simulink model "RBDmodel_unprotected"  (R2023a)
settings: Solver=ode15s  StartTime=0.0  StopTime=10  FixedStep=0.0001  RelTol=1e-3  AbsTol=1e-3  EnableMultiTasking=on
model workspace (MAT data in the model file):
  C_Gimbal = 0.1
  C_IAP = 0.01
  IAP_Pa = 0
  K_Gimbal = 0
  K_IAP = 0
  Left_EO = 0
  Left_IO = 0
  Left_MF = 0
  Left_RA = 0
  Moment_AR = 0
  Moment_FE = 7.5
  Moment_LB = 0
  Right_EO = 0
  Right_IO = 0
  Right_MF = 0
  Right_RA = 0
  a = 1
  b = 1
  muscle_color = [0 0 1]
  muscle_radius = 1
undefined symbols (not defined in the file): X, Y, Z
libraries: nesl_utility x346, sm_lib x329, simulink_extras x33, checkpacklib x3, simulink x1
(part 1 of 13)
settings Model: PacingRate=0.110000  Creator=Siril TD  LastModifiedBy=siril
settings SolverCC: ZeroCrossAlgorithm=Adaptive  AutoInsertRateTranBlk=on
settings DataIOCC: LimitDataPoints=on  MaxDataPoints=50000  ReturnWorkspaceOutputsName=SDOSimTest_Log
settings OptimizationCC: LifeSpan=inf
settings DebuggingCC: IgnoredZcDiagnostic=none  UnconnectedInputMsg=warning  UnconnectedOutputMsg=warning  UnconnectedLineMsg=warning  AllowSymbolicDim=off  SFUnexpectedBacktrackingDiag=warning  SFNoUnconditionalDefaultTransitionDiag=warning  SFExecutionAtInitializationDiag=none  ArithmeticOperatorsInVariantConditions=warning
settings ModelReferenceCC: EnableRefExpFcnMdlSchedulingChecks=on
settings SFSimCC: SimUseLocalCustomCode=off  CustomCodeUndefinedFunction=UseInterfaceOnly
settings RTWCC: RTWUseLocalCustomCode=off  DLArmComputeVersion=19.05
settings CodeAppCC: StateflowObjectComments=on
settings GRTTargetCC: TargetLangStandard=C89/C90 (ANSI)
settings ConfigComp: CovMetricSettings=dw  CovSaveCumulativeToWorkspaceVar=on  CovSaveSingleToWorkspaceVar=on  CovExternalEMLEnable=off  CovSFcnEnable=off
settings SimscapeCC: SimscapeLogType=all  SimscapeLogSimulationStatistics=on  SimscapeLogDataHistory=10000

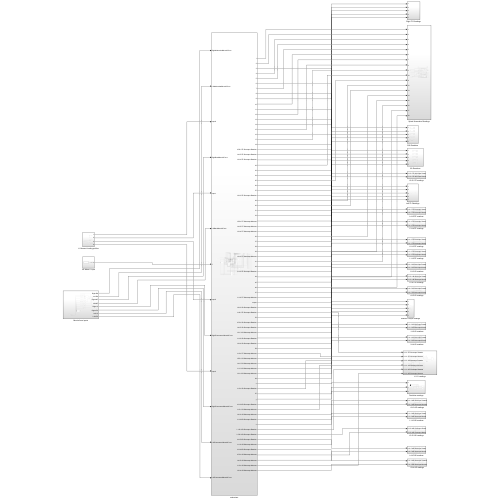
[thumbnail: Simulink's stored preview of the top-level diagram]
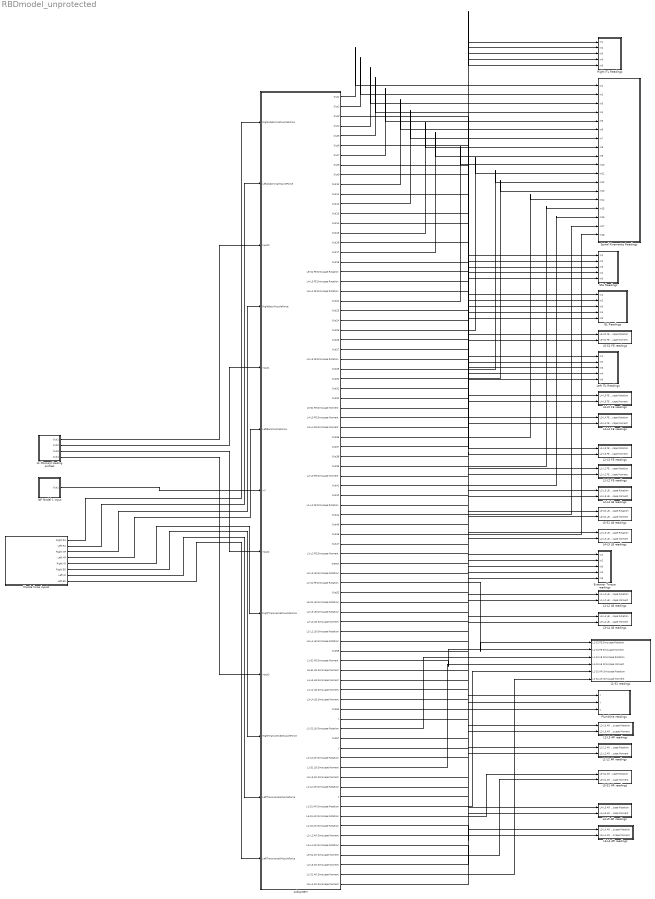
== system RBDmodel_unprotected ==
  Extensor Torque readings : Subsystem
  IAP Model 1 input : Subsystem
  ISL Readings : Subsystem
  L1 Moment loading profiles : Subsystem
  L1-L2 AR readings : Subsystem
  L1-L2 FE readings : Subsystem
  L1-L2 LB readings : Subsystem
  L1-S1 readings : Subsystem
  L2-L3 AR readings : Subsystem
  L2-L3 FE readings : Subsystem
  L2-L3 LB readings : Subsystem
  L3-L4 AR readings : Subsystem
  L3-L4 FE readings : Subsystem
  L3-L4 LB readings : Subsystem
  L4-L5 AR readings : Subsystem
  L4-L5 FE readings : Subsystem
  L4-L5 LB readings : Subsystem
  L5-S1 AR readings : Subsystem
  L5-S1 FE readings : Subsystem
  L5-S1 LB readings : Subsystem
  Left ITL Readings : Subsystem
  Muscle force inputs : Subsystem
  Plumbline readings : Subsystem
  Right ITL Readings : Subsystem
  SSL Readings : Subsystem
  Spinal Kinematics Readings : Subsystem
  subsystem : Subsystem
  wires:
  Muscle force inputs/1(Right RA) -> subsystem/1(RightAbdominalMuscleForce)
  Muscle force inputs/2(Left RA) -> subsystem/2(LeftAbdominalMuscleForce)
  L1 Moment loading profiles/1(Out1) -> subsystem/3(input0)
  Muscle force inputs/3(Right MF) -> subsystem/4(RightBackMuscleForce)
  L1 Moment loading profiles/2(Out2) -> subsystem/5(input1)
  Muscle force inputs/4(Left MF) -> subsystem/6(LeftBackMuscleForce)
  IAP Model 1 input/1(Out1) -> subsystem/7(In7)
  L1 Moment loading profiles/3(Out3) -> subsystem/8(input2)
  Muscle force inputs/5(Right IO) -> subsystem/9(RightTransverse1MuscleForce)
  L1 Moment loading profiles/4(Out4) -> subsystem/10(input3)
  Muscle force inputs/6(Right EO) -> subsystem/11(RightTransverse2MuscleForce)
  Muscle force inputs/7(Left IO) -> subsystem/12(LeftTransverse1MuscleForce)
  Muscle force inputs/8(Left EO) -> subsystem/13(LeftTransverse2MuscleForce)
  subsystem/1(Out1) -> Spinal Kinematics Readings/1(In1)
  subsystem/2(Out2) -> Spinal Kinematics Readings/2(In2)
  subsystem/3(Out3) -> ISL Readings/1(In1)
  subsystem/4(Out4) -> Spinal Kinematics Readings/3(In3)
  subsystem/5(Out5) -> Spinal Kinematics Readings/4(In4)
  subsystem/6(Out6) -> SSL Readings/1(In1)
  subsystem/7(Out7) -> Spinal Kinematics Readings/5(In5)
  subsystem/8(Out8) -> Left ITL Readings/1(In1)
  subsystem/9(Out9) -> Right ITL Readings/1(In1)
  subsystem/10(Out10) -> Spinal Kinematics Readings/6(In6)
  subsystem/11(Out11) -> ISL Readings/2(In2)
  subsystem/12(Out12) -> Spinal Kinematics Readings/7(In7)
  subsystem/13(Out13) -> SSL Readings/2(In2)
  subsystem/14(Out14) -> Right ITL Readings/2(In2)
  subsystem/15(Out15) -> Spinal Kinematics Readings/8(In8)
  subsystem/16(Out16) -> Left ITL Readings/2(In2)
  subsystem/17(Out17) -> Spinal Kinematics Readings/9(In9)
  subsystem/18(Out18) -> Right ITL Readings/3(In3)
  subsystem/19(L5-S1 FE Simscape Rotation) -> L5-S1 FE readings/1(L5-S1 FE Simscape Rotation)
  subsystem/20(L4-L5 FE Simscape Rotation) -> L4-L5 FE readings/1(L4-L5 FE Simscape Rotation)
  subsystem/21(L3-L4 FE Simscape Rotation) -> L3-L4 FE readings/1(L3-L4 FE Simscape Rotation)
  subsystem/22(Out22) -> Spinal Kinematics Readings/10(In10)
  subsystem/23(Out23) -> ISL Readings/3(In3)
  subsystem/24(Out24) -> SSL Readings/3(In3)
  subsystem/25(Out25) -> Spinal Kinematics Readings/11(In11)
  subsystem/26(Out26) -> Left ITL Readings/3(In3)
  subsystem/27(Out27) -> Right ITL Readings/4(In4)
  subsystem/28(L2-L3 FE Simscape Rotation) -> L2-L3 FE readings/1(L2-L3 FE Simscape Rotation)
  subsystem/29(Out29) -> Spinal Kinematics Readings/12(In12)
  subsystem/30(Out30) -> Spinal Kinematics Readings/13(In13)
  subsystem/31(Out31) -> SSL Readings/4(In4)
  subsystem/32(Out32) -> Right ITL Readings/5(In5)
  subsystem/33(L5-S1 FE Simscape Moment) -> L5-S1 FE readings/2(L5-S1 FE Simscape Moment)
  subsystem/34(L4-L5 FE Simscape Moment) -> L4-L5 FE readings/2(L4-L5 FE Simscape Moment)
  subsystem/35(L3-L4 FE Simscape Moment) -> L3-L4 FE readings/2(L3-L4 FE Simscape Moment)
  subsystem/36(Out36) -> Spinal Kinematics Readings/14(In14)
  subsystem/37(Out37) -> ISL Readings/4(In4)
  subsystem/38(Out38) -> Left ITL Readings/4(In4)
  subsystem/39(Out39) -> Spinal Kinematics Readings/15(In15)
  subsystem/40(L2-L3 FE Simscape Moment) -> L2-L3 FE readings/2(L2-L3 FE Simscape Moment)
  subsystem/41(Out41) -> Spinal Kinematics Readings/16(In16)
  subsystem/42(Out42) -> SSL Readings/5(In5)
  subsystem/43(L1-L2 FE Simscape Rotation) -> L1-L2 FE readings/1(L1-L2 FE Simscape Rotation)
  subsystem/44(Out44) -> Spinal Kinematics Readings/17(In17)
  subsystem/45(Out45) -> Left ITL Readings/5(In5)
  subsystem/46(Out46) -> Spinal Kinematics Readings/18(In18)
  subsystem/47(Out47) -> ISL Readings/5(In5)
  subsystem/48(L1-L2 FE Simscape Moment) -> L1-L2 FE readings/2(L1-L2 FE Simscape Moment)
  subsystem/49(output) -> Extensor Torque readings/1(In1)
  subsystem/50(L2-L3 LB Simscape Rotation) -> L2-L3 LB readings/1(L2-L3 LB Simscape Rotation)
  subsystem/51(L1-S1 FE Simscape Rotation) -> L1-S1 readings/1(L1-S1 FE Simscape Rotation)
  subsystem/52(Out52) -> Extensor Torque readings/2(In2)
  subsystem/53(L5-S1 LB Simscape Rotation) -> L5-S1 LB readings/1(L5-S1 LB Simscape Rotation)
  subsystem/54(L4-L5 LB Simscape Rotation) -> L4-L5 LB readings/1(L4-L5 LB Simscape Rotation)
  subsystem/55(L2-L3 LB Simscape Moment) -> L2-L3 LB readings/2(L2-L3 LB Simscape Moment)
  subsystem/56(L1-L2 LB Simscape Rotation) -> L1-L2 LB readings/1(L1-L2 LB Simscape Rotation)
  subsystem/57(L3-L4 LB Simscape Rotation) -> L3-L4 LB readings/1(L3-L4 LB Simscape Rotation)
  subsystem/58(Out58) -> Extensor Torque readings/3(In3)
  subsystem/59(L1-S1 FE Simscape Moment) -> L1-S1 readings/2(L1-S1 FE Simscape Moment)
  subsystem/60(L5-S1 LB Simscape Moment) -> L5-S1 LB readings/2(L5-S1 LB Simscape Moment)
  subsystem/61(L4-L5 LB Simscape Moment) -> L4-L5 LB readings/2(L4-L5 LB Simscape Moment)
  subsystem/62(L1-L2 LB Simscape Moment) -> L1-L2 LB readings/2(L1-L2 LB Simscape Moment)
  subsystem/63(L3-L4 LB Simscape Moment) -> L3-L4 LB readings/2(L3-L4 LB Simscape Moment)
  subsystem/64(Out64) -> Extensor Torque readings/4(In4)
  subsystem/65(x) -> Plumbline readings/1(x)
  subsystem/66(L1-S1 LB Simscape Rotation) -> L1-S1 readings/3(L1-S1 LB Simscape Rotation)
  subsystem/67(Out67) -> Extensor Torque readings/5(In5)
  subsystem/68(y) -> Plumbline readings/2(y)
  subsystem/69(L2-L3 AR Simscape Rotation) -> L2-L3 AR readings/1(L2-L3 AR Simscape Rotation)
  subsystem/70(L1-S1 LB Simscape Moment) -> L1-S1 readings/4(L1-S1 LB Simscape Moment)
  subsystem/71(L2-L3 AR Simscape Moment) -> L2-L3 AR readings/2(L2-L3 AR Simscape Moment)
  subsystem/72(L1-L2 AR Simscape Rotation) -> L1-L2 AR readings/1(L1-L2 AR Simscape Rotation)
  subsystem/73(z) -> Plumbline readings/3(z)
  subsystem/74(L1-S1 AR Simscape Rotation) -> L1-S1 readings/5(L1-S1 AR Simscape Rotation)
  subsystem/75(L5-S1 AR Simscape Rotation) -> L5-S1 AR readings/1(L5-S1 AR Simscape Rotation)
  subsystem/76(L4-L5 AR Simscape Rotation) -> L4-L5 AR readings/1(L4-L5 AR Simscape Rotation)
  subsystem/77(L1-L2 AR Simscape Moment) -> L1-L2 AR readings/2(L1-L2 AR Simscape Moment)
  subsystem/78(L3-L4 AR Simscape Rotation) -> L3-L4 AR readings/1(L3-L4 AR Simscape Rotation)
  subsystem/79(L5-S1 AR Simscape Moment) -> L5-S1 AR readings/2(L5-S1 AR Simscape Moment)
  subsystem/80(L4-L5 AR Simscape Moment) -> L4-L5 AR readings/2(L4-L5 AR Simscape Moment)
  subsystem/81(L1-S1 AR Simscape Moment) -> L1-S1 readings/6(L1-S1 AR Simscape Moment)
  subsystem/82(L3-L4 AR Simscape Moment) -> L3-L4 AR readings/2(L3-L4 AR Simscape Moment)

== system RBDmodel_unprotected/Extensor Torque readings ==
  In1 : Inport
  In2 : Inport  Port=2
  In3 : Inport  Port=3
  In4 : Inport  Port=4
  In5 : Inport  Port=5
  Display{,1..4} (5 alike) : Display
      settings: Decimation=2
  Gain{9,11..14} (5 alike) : Gain
  IAP Extensor Torque at L1-L2 : Scope
  IAP Extensor Torque at L2-L3 (reported) : Scope
  IAP Extensor Torque at L3-L4 : Scope
  IAP Extensor Torque at L4-L5 : Scope
  IAP Extensor Torque at L5-S1 : Scope
  wires:
  Gain11/1 -> Display1/1
  Gain9/1 -> Display/1
  In5/1 -> Gain14/1, IAP Extensor Torque at L5-S1/1
  In2/1 -> Gain9/1, IAP Extensor Torque at L2-L3 (reported)/1
  Gain12/1 -> Display2/1
  In4/1 -> Gain13/1, IAP Extensor Torque at L4-L5/1
  In3/1 -> Gain12/1, IAP Extensor Torque at L3-L4/1
  Gain13/1 -> Display3/1
  In1/1 -> Gain11/1, IAP Extensor Torque at L1-L2/1
  Gain14/1 -> Display4/1

== system RBDmodel_unprotected/IAP Model 1 input ==
  Constant96 : Constant  Value=IAP_Pa
  Out1 : Outport
  wires:
  Constant96/1 -> Out1/1

== system RBDmodel_unprotected/ISL Readings ==
  In1 : Inport
  In2 : Inport  Port=2
  In3 : Inport  Port=3
  In4 : Inport  Port=4
  In5 : Inport  Port=5
  L1-L2 ISL force : Scope
  L2-L3 ISL force : Scope
  L3-L4 ISL force : Scope
  L4-L5 ISL force : Scope
  L5-S1 ISL force : Scope
  wires:
  In4/1 -> L5-S1 ISL force/1
  In2/1 -> L2-L3 ISL force/1
  In1/1 -> L1-L2 ISL force/1
  In3/1 -> L3-L4 ISL force/1
  In5/1 -> L4-L5 ISL force/1

== system RBDmodel_unprotected/L1 Moment loading profiles ==
  Gain10 : Gain  Gain=-1
  Horizontal force at T1 : simulink/Sources/Ramp  slope=0  start=0  InitialOutput=0
  Moment_AR : Sin  Amplitude=Moment_AR  SampleTime=0
  Moment_FE : Sin  Amplitude=-Moment_FE  SampleTime=0
  Moment_LB : Sin  Amplitude=-Moment_LB  SampleTime=0
  Scope2 : Scope
  Out1 : Outport
  Out2 : Outport  Port=2
  Out3 : Outport  Port=3
  Out4 : Outport  Port=4
  wires:
  Gain10/1 -> Scope2/1
  Horizontal force at T1/1 -> Out4/1
  Moment_LB/1 -> Out2/1
  Moment_AR/1 -> Out1/1
  Moment_FE/1 -> Gain10/1, Out3/1

== system RBDmodel_unprotected/L1-L2 AR readings ==
  L1-L2 AR Simscape Rotation : Inport
  L1-L2 AR Simscape Moment : Inport  Port=2
  L1-L2 AR Moment : Scope
  L1-L2 AR Rotation : Scope
  L1-L2 AR Simscape : Record  FileSettingsInternal="{\"entries\":[{\"content\":{\"excelSettings\":{\"content\":{},\"type\":\"Streamout.ExcelSettings\"}},\"type\":\"Streamout.FileSettingStorage\",\"uuid\":\"0b07cbdd-b916-43fe-bdd8-9a10c94332a9\"}],\"packageUris\":[\"http://schema.mathworks.com/mf0/streamout_blocks/R2020a\"],\"version\":\"1.0\"}"  Layout=[1 1]  SignalsInternal="{\"entries\":[{\"content\":{\"signals\":[{\"content\":{\"blockPath\":[\"RBDmodel/L1-L2 AR readings/L1-L2 AR Simscape\"],\"dimensions\":[1],\"domain\":\"RBDmodel/L1-L2 AR readings/L1-L2 AR Simscape\",\"lineColor\":\"#64d413\",\"port\":1,\"sid\":[\"\"],\"signalID\":1824,\"signalName\":\"L1-L2 AR Simscape Rotation\"},\"type\":\"RecordBlkView.Signal\",\"uuid\":\"c0e7ae7a-cc90-4b18-a108-b90de0d6dcb7\"},{\"content\":{\"blockPath\":[\"RBDmodel/L1-L2 AR readings/L1-L2 AR Simscape\"],\"dimensions\":[1],\"domain\":\"RBDmodel/L1-L2 AR readings/L1-L2 AR Simscape\",\"lineColor\":\"#ff13a6\",\"port\":2,\"sid\":[\"\"],\"signalID\":1828,\"signalName\":\"L1-L2 AR Simscape Moment\"},\"type\":\"RecordBlkView.Signal\",\"uuid\":\"6882256b-2454-4389-9940-6dc4d3647226\"}]},\"type\":\"RecordBlkView.InputSignals\",\"uuid\":\"5ddb2381-f46e-4a36-855d-7c42eb17c628\"}],\"packageUris\":[\"http://schema.mathworks.com/mf0/streamout_blocks/R2020a\"],\"version\":\"1.0\"}"  VisualizationBindings="{\"xyplotplugin\":{\"info\":[{\"series\":[],\"subplotID\":1}]}}"  CompatibilityTag=XY
  wires:
  L1-L2 AR Simscape Rotation/1 -> L1-L2 AR Simscape/1, L1-L2 AR Rotation/1
  L1-L2 AR Simscape Moment/1 -> L1-L2 AR Simscape/2, L1-L2 AR Moment/1

== system RBDmodel_unprotected/L1-L2 FE readings ==
  L1-L2 FE Simscape Rotation : Inport
  L1-L2 FE Simscape Moment : Inport  Port=2
  L1-L2 FE Moment : Scope
  L1-L2 FE Rotation : Scope
  L1-L2 FE Simscape : Record  FileSettingsInternal="{\"entries\":[{\"content\":{\"excelSettings\":{\"content\":{},\"type\":\"Streamout.ExcelSettings\"}},\"type\":\"Streamout.FileSettingStorage\",\"uuid\":\"e81f3c3b-fdd2-4aa4-ae18-e10074030446\"}],\"packageUris\":[\"http://schema.mathworks.com/mf0/streamout_blocks/R2020a\"],\"version\":\"1.0\"}"  Layout=[1 1]  SignalsInternal="{\"entries\":[{\"content\":{\"signals\":[{\"content\":{\"blockPath\":[\"RBDmodel/L1-L2 FE readings/L1-L2 FE Simscape\"],\"dimensions\":[1],\"domain\":\"RBDmodel/L1-L2 FE readings/L1-L2 FE Simscape\",\"lineColor\":\"#fe330a\",\"port\":1,\"sid\":[\"\"],\"signalID\":1832,\"signalName\":\"L1-L2 FE Simscape Rotation\"},\"type\":\"RecordBlkView.Signal\",\"uuid\":\"4f83da81-b97e-4b8c-8069-88fdcce7431f\"},{\"content\":{\"blockPath\":[\"RBDmodel/L1-L2 FE readings/L1-L2 FE Simscape\"],\"dimensions\":[1],\"domain\":\"RBDmodel/L1-L2 FE readings/L1-L2 FE Simscape\",\"lineColor\":\"#22b573\",\"port\":2,\"sid\":[\"\"],\"signalID\":1836,\"signalName\":\"L1-L2 FE Simscape Moment\"},\"type\":\"RecordBlkView.Signal\",\"uuid\":\"63cb8a53-fa8c-4023-a5b8-adb7ee7d6e97\"}]},\"type\":\"RecordBlkView.InputSignals\",\"uuid\":\"c644fd37-6f36-41c8-98c8-0c3b16469eb2\"}],\"packageUris\":[\"http://schema.mathworks.com/mf0/streamout_blocks/R2020a\"],\"version\":\"1.0\"}"  VisualizationBindings="{\"xyplotplugin\":{\"info\":[{\"series\":[],\"subplotID\":1}]}}"  CompatibilityTag=XY
  wires:
  L1-L2 FE Simscape Rotation/1 -> L1-L2 FE Simscape/1, L1-L2 FE Rotation/1
  L1-L2 FE Simscape Moment/1 -> L1-L2 FE Simscape/2, L1-L2 FE Moment/1

== system RBDmodel_unprotected/L1-L2 LB readings ==
  L1-L2 LB Simscape Rotation : Inport
  L1-L2 LB Simscape Moment : Inport  Port=2
  L1-L2 LB Moment : Scope
  L1-L2 LB Rotation : Scope
  L1-L2 LB Simscape : Record  FileSettingsInternal="{\"entries\":[{\"content\":{\"excelSettings\":{\"content\":{},\"type\":\"Streamout.ExcelSettings\"}},\"type\":\"Streamout.FileSettingStorage\",\"uuid\":\"af119469-5f93-400d-9cae-3a354b70e1a3\"}],\"packageUris\":[\"http://schema.mathworks.com/mf0/streamout_blocks/R2020a\"],\"version\":\"1.0\"}"  Layout=[1 1]  SignalsInternal="{\"entries\":[{\"content\":{\"signals\":[{\"content\":{\"blockPath\":[\"RBDmodel/L1-L2 LB readings/L1-L2 LB Simscape\"],\"dimensions\":[1],\"domain\":\"RBDmodel/L1-L2 LB readings/L1-L2 LB Simscape\",\"lineColor\":\"#0072bd\",\"port\":1,\"sid\":[\"\"],\"signalID\":1840,\"signalName\":\"L1-L2 LB Simscape Rotation\"},\"type\":\"RecordBlkView.Signal\",\"uuid\":\"793cf4fb-6b0b-4fcd-9071-091689e68879\"},{\"content\":{\"blockPath\":[\"RBDmodel/L1-L2 LB readings/L1-L2 LB Simscape\"],\"dimensions\":[1],\"domain\":\"RBDmodel/L1-L2 LB readings/L1-L2 LB Simscape\",\"lineColor\":\"#d95319\",\"port\":2,\"sid\":[\"\"],\"signalID\":1844,\"signalName\":\"L1-L2 LB Simscape Moment\"},\"type\":\"RecordBlkView.Signal\",\"uuid\":\"9aa3d4d4-c80e-4f4b-87d4-792e86b33535\"}]},\"type\":\"RecordBlkView.InputSignals\",\"uuid\":\"32d59bc1-78ac-4b25-82dd-58f854734bb6\"}],\"packageUris\":[\"http://schema.mathworks.com/mf0/streamout_blocks/R2020a\"],\"version\":\"1.0\"}"  VisualizationBindings="{\"xyplotplugin\":{\"info\":[{\"series\":[],\"subplotID\":1}]}}"  CompatibilityTag=XY
  wires:
  L1-L2 LB Simscape Moment/1 -> L1-L2 LB Simscape/2, L1-L2 LB Moment/1
  L1-L2 LB Simscape Rotation/1 -> L1-L2 LB Simscape/1, L1-L2 LB Rotation/1

== system RBDmodel_unprotected/L1-S1 readings ==
  L1-S1 FE Simscape Rotation : Inport
  L1-S1 FE Simscape Moment : Inport  Port=2
  L1-S1 LB Simscape Rotation : Inport  Port=3
  L1-S1 LB Simscape Moment : Inport  Port=4
  L1-S1 AR Simscape Rotation : Inport  Port=5
  L1-S1 AR Simscape Moment : Inport  Port=6
  Check Flexion Angle : checkpacklib/Check Custom Bounds  InstantiateOnLoad=on  enabled=off  stopWhenAssertionFail=off  export=off  ViewDlgPos=[100 200 510 390]  OpenViewOnLoad=off  LaunchViewOnOpen=off  TimeUnits=seconds  EnableUpperBound=on  UpperBoundTimes=[5 10]  UpperBoundAmplitudes=[51 51];  EnableLowerBound=on  LowerBoundTimes=[6 10]  LowerBoundAmplitudes=[49 49];
      settings: LibrarySourceBlock=sdolib/Signal Constraints/Check Custom Bounds
  L1-S1 AR Rotation : Scope
  L1-S1 AR Simscape : Record  FileSettingsInternal="{\"entries\":[{\"content\":{\"excelSettings\":{\"content\":{},\"type\":\"Streamout.ExcelSettings\"}},\"type\":\"Streamout.FileSettingStorage\",\"uuid\":\"8b435ecc-68fb-4417-98fb-e21cddb23a2a\"}],\"packageUris\":[\"http://schema.mathworks.com/mf0/streamout_blocks/R2020a\"],\"version\":\"1.0\"}"  Layout=[1 1]  SignalsInternal="{\"entries\":[{\"content\":{\"signals\":[{\"content\":{\"blockPath\":[\"RBDmodel/L1-S1 readings/L1-S1 AR Simscape\"],\"dimensions\":[1,1],\"domain\":\"RBDmodel/L1-S1 readings/L1-S1 AR Simscape\",\"lineColor\":\"#77ac30\",\"port\":1,\"sid\":[\"\"],\"signalID\":1856,\"signalName\":\"L1-S1 AR Simscape Rotation\"},\"type\":\"RecordBlkView.Signal\",\"uuid\":\"d687226c-a4af-4711-b276-2389fb4ab0b8\"},{\"content\":{\"blockPath\":[\"RBDmodel/L1-S1 readings/L1-S1 AR Simscape\"],\"dimensions\":[1],\"domain\":\"RBDmodel/L1-S1 readings/L1-S1 AR Simscape\",\"lineColor\":\"#4dbeee\",\"port\":2,\"sid\":[\"\"],\"signalID\":1860,\"signalName\":\"L1-S1 AR Simscape Moment\"},\"type\":\"RecordBlkView.Signal\",\"uuid\":\"3fcdb553-42d1-479c-9858-cf9711b04ff0\"}]},\"type\":\"RecordBlkView.InputSignals\",\"uuid\":\"f7dab850-abf6-4c98-91ce-33abad572001\"}],\"packageUris\":[\"http://schema.mathworks.com/mf0/streamout_blocks/R2020a\"],\"version\":\"1.0\"}"  VisualizationBindings="{\"xyplotplugin\":{\"info\":[{\"series\":[],\"subplotID\":1}]}}"  CompatibilityTag=XY
  L1-S1 AR when LB loading : Record  FileSettingsInternal="{\"entries\":[{\"content\":{\"excelSettings\":{\"content\":{},\"type\":\"Streamout.ExcelSettings\"}},\"type\":\"Streamout.FileSettingStorage\",\"uuid\":\"3646d6ae-8fa2-41c0-8a30-b8d0ca000973\"}],\"packageUris\":[\"http://schema.mathworks.com/mf0/streamout_blocks/R2020a\"],\"version\":\"1.0\"}"  Layout=[1 1]  SignalsInternal="{\"entries\":[{\"content\":{\"signals\":[{\"content\":{\"blockPath\":[\"RBDmodel/L1-S1 readings/L1-S1 AR when LB loading\"],\"dimensions\":[1,1],\"domain\":\"RBDmodel/L1-S1 readings/L1-S1 AR when LB loading\",\"lineColor\":\"#a2142f\",\"port\":1,\"sid\":[\"\"],\"signalID\":1864,\"signalName\":\"L1-S1 AR Simscape Rotation\"},\"type\":\"RecordBlkView.Signal\",\"uuid\":\"555ee46b-423f-4f6b-b8d0-63163656811b\"},{\"content\":{\"blockPath\":[\"RBDmodel/L1-S1 readings/L1-S1 AR when LB loading\"],\"dimensions\":[1],\"domain\":\"RBDmodel/L1-S1 readings/L1-S1 AR when LB loading\",\"lineColor\":\"#139fff\",\"port\":2,\"sid\":[\"\"],\"signalID\":1868,\"signalName\":\"L1-S1 LB Simscape Moment\"},\"type\":\"RecordBlkView.Signal\",\"uuid\":\"6d47c88b-b77f-449c-b8c2-23ad0cb1820e\"}]},\"type\":\"RecordBlkView.InputSignals\",\"uuid\":\"ac151119-312c-446c-9fd5-09a961120854\"}],\"packageUris\":[\"http://schema.mathworks.com/mf0/streamout_blocks/R2020a\"],\"version\":\"1.0\"}"  VisualizationBindings="{\"xyplotplugin\":{\"info\":[{\"series\":[],\"subplotID\":1}]}}"  CompatibilityTag=XY
  L1-S1 FE Rotation : Scope
  L1-S1 FE Simscape : Record  FileSettingsInternal="{\"entries\":[{\"content\":{\"excelSettings\":{\"content\":{},\"type\":\"Streamout.ExcelSettings\"}},\"type\":\"Streamout.FileSettingStorage\",\"uuid\":\"60c6a6dc-6af9-4681-aa25-453a1e3fb2e7\"}],\"packageUris\":[\"http://schema.mathworks.com/mf0/streamout_blocks/R2020a\"],\"version\":\"1.0\"}"  Layout=[1 1]  SignalsInternal="{\"entries\":[{\"content\":{\"signals\":[{\"content\":{\"blockPath\":[\"RBDmodel/L1-S1 readings/L1-S1 FE Simscape\"],\"dimensions\":[1,1],\"domain\":\"RBDmodel/L1-S1 readings/L1-S1 FE Simscape\",\"lineColor\":\"#edb120\",\"plots\":[1],\"port\":1,\"sid\":[\"\"],\"signalID\":1848,\"signalName\":\"L1-S1 FE Simscape Rotation\"},\"type\":\"RecordBlkView.Signal\",\"uuid\":\"1cfc74e7-ce87-4fa0-a069-ab785adc6ac7\"},{\"content\":{\"blockPath\":[\"RBDmodel/L1-S1 readings/L1-S1 FE Simscape\"],\"dimensions\":[1],\"domain\":\"RBDmodel/L1-S1 readings/L1-S1 FE Simscape\",\"lineColor\":\"#7e2f8e\",\"plots\":[1],\"port\":2,\"sid\":[\"\"],\"signalID\":1852,\"signalName\":\"L1-S1 FE Simscape Moment\"},\"type\":\"RecordBlkView.Signal\",\"uuid\":\"f9ae6916-9979-4bfa-876b-8483df570262\"}]},\"type\":\"RecordBlkView.InputSignals\",\"uuid\":\"b7057824-dcfb-47a1-9c18-344bdabb32be\"}],\"packageUris\":[\"http://schema.mathworks.com/mf0/streamout_blocks/R2020a\"],\"version\":\"1.0\"}"  VisualizationBindings="{\"xyplotplugin\":{\"info\":[{\"series\":[{\"bindingParametersList\":[{\"parameter\":\"X-Axis\",\"signalID\":1852,\"signalName\":\"L1-S1 FE Simscape Moment\"},{\"parameter\":\"Y-Axis\",\"signalID\":1848,\"signalName\":\"L1-S1 FE Simscape Rotation\"}],\"seriesID\":21130}],\"subplotID\":1}]}}"  CompatibilityTag=XY
  L1-S1 LB Rotation : Scope
  L1-S1 LB Simscape : Record  FileSettingsInternal="{\"entries\":[{\"content\":{\"excelSettings\":{\"content\":{},\"type\":\"Streamout.ExcelSettings\"}},\"type\":\"Streamout.FileSettingStorage\",\"uuid\":\"12ee75cc-314c-466c-ae00-c939b030dc7e\"}],\"packageUris\":[\"http://schema.mathworks.com/mf0/streamout_blocks/R2020a\"],\"version\":\"1.0\"}"  Layout=[1 1]  SignalsInternal="{\"entries\":[{\"content\":{\"signals\":[{\"content\":{\"blockPath\":[\"RBDmodel/L1-S1 readings/L1-S1 LB Simscape\"],\"dimensions\":[1,1],\"domain\":\"RBDmodel/L1-S1 readings/L1-S1 LB Simscape\",\"lineColor\":\"#ff6929\",\"port\":1,\"sid\":[\"\"],\"signalID\":1872,\"signalName\":\"L1-S1 LB Simscape Rotation\"},\"type\":\"RecordBlkView.Signal\",\"uuid\":\"51ca59bd-28ce-458d-8754-f1bc6e03cbdb\"},{\"content\":{\"blockPath\":[\"RBDmodel/L1-S1 readings/L1-S1 LB Simscape\"],\"dimensions\":[1],\"domain\":\"RBDmodel/L1-S1 readings/L1-S1 LB Simscape\",\"lineColor\":\"#b746ff\",\"port\":2,\"sid\":[\"\"],\"signalID\":1876,\"signalName\":\"L1-S1 LB Simscape Moment\"},\"type\":\"RecordBlkView.Signal\",\"uuid\":\"686fd1a9-4131-4eb8-9c6b-f244a8bb1047\"}]},\"type\":\"RecordBlkView.InputSignals\",\"uuid\":\"ee63b32a-13a3-429f-9975-3a8057803029\"}],\"packageUris\":[\"http://schema.mathworks.com/mf0/streamout_blocks/R2020a\"],\"version\":\"1.0\"}"  VisualizationBindings="{\"xyplotplugin\":{\"info\":[{\"series\":[],\"subplotID\":1}]}}"  CompatibilityTag=XY
  wires:
  L1-S1 LB Simscape Rotation/1 -> L1-S1 LB Simscape/1, L1-S1 LB Rotation/1
  L1-S1 FE Simscape Rotation/1 -> Check Flexion Angle/1, L1-S1 FE Rotation/1, L1-S1 FE Simscape/1
  L1-S1 AR Simscape Rotation/1 -> L1-S1 AR when LB loading/1, L1-S1 AR Rotation/1, L1-S1 AR Simscape/1
  L1-S1 LB Simscape Moment/1 -> L1-S1 LB Simscape/2, L1-S1 AR when LB loading/2
  L1-S1 FE Simscape Moment/1 -> L1-S1 FE Simscape/2
  L1-S1 AR Simscape Moment/1 -> L1-S1 AR Simscape/2

== system RBDmodel_unprotected/L2-L3 AR readings ==
  L2-L3 AR Simscape Rotation : Inport
  L2-L3 AR Simscape Moment : Inport  Port=2
  L2-L3 AR Moment : Scope
  L2-L3 AR Rotation : Scope
  L2-L3 AR Simscape : Record  FileSettingsInternal="{\"entries\":[{\"content\":{\"excelSettings\":{\"content\":{},\"type\":\"Streamout.ExcelSettings\"}},\"type\":\"Streamout.FileSettingStorage\",\"uuid\":\"b562e67b-ebcf-4506-bf51-7643245480cd\"}],\"packageUris\":[\"http://schema.mathworks.com/mf0/streamout_blocks/R2020a\"],\"version\":\"1.0\"}"  Layout=[1 1]  SignalsInternal="{\"entries\":[{\"content\":{\"signals\":[{\"content\":{\"blockPath\":[\"RBDmodel/L2-L3 AR readings/L2-L3 AR Simscape\"],\"dimensions\":[1],\"domain\":\"RBDmodel/L2-L3 AR readings/L2-L3 AR Simscape\",\"lineColor\":\"#64d413\",\"port\":1,\"sid\":[\"\"],\"signalID\":1880,\"signalName\":\"L2-L3 AR Simscape Rotation\"},\"type\":\"RecordBlkView.Signal\",\"uuid\":\"b50a5c46-7e05-4311-93ea-b9366bb19537\"},{\"content\":{\"blockPath\":[\"RBDmodel/L2-L3 AR readings/L2-L3 AR Simscape\"],\"dimensions\":[1],\"domain\":\"RBDmodel/L2-L3 AR readings/L2-L3 AR Simscape\",\"lineColor\":\"#ff13a6\",\"port\":2,\"sid\":[\"\"],\"signalID\":1884,\"signalName\":\"L2-L3 AR Simscape Moment\"},\"type\":\"RecordBlkView.Signal\",\"uuid\":\"312e3dd4-a8fc-4c58-b11f-fab1914326f6\"}]},\"type\":\"RecordBlkView.InputSignals\",\"uuid\":\"88feaefb-60e9-4aed-858f-55149aa6adeb\"}],\"packageUris\":[\"http://schema.mathworks.com/mf0/streamout_blocks/R2020a\"],\"version\":\"1.0\"}"  VisualizationBindings="{\"xyplotplugin\":{\"info\":[{\"series\":[],\"subplotID\":1}]}}"  CompatibilityTag=XY
  wires:
  L2-L3 AR Simscape Rotation/1 -> L2-L3 AR Simscape/1, L2-L3 AR Rotation/1
  L2-L3 AR Simscape Moment/1 -> L2-L3 AR Simscape/2, L2-L3 AR Moment/1

== system RBDmodel_unprotected/L2-L3 FE readings ==
  L2-L3 FE Simscape Rotation : Inport
  L2-L3 FE Simscape Moment : Inport  Port=2
  L2-L3 FE Moment : Scope
  L2-L3 FE Rotation : Scope
  L2-L3 FE Simscape : Record  FileSettingsInternal="{\"entries\":[{\"content\":{\"excelSettings\":{\"content\":{},\"type\":\"Streamout.ExcelSettings\"}},\"type\":\"Streamout.FileSettingStorage\",\"uuid\":\"60a6d423-89c4-4085-b0aa-020154b09243\"}],\"packageUris\":[\"http://schema.mathworks.com/mf0/streamout_blocks/R2020a\"],\"version\":\"1.0\"}"  Layout=[1 1]  SignalsInternal="{\"entries\":[{\"content\":{\"signals\":[{\"content\":{\"blockPath\":[\"RBDmodel/L2-L3 FE readings/L2-L3 FE Simscape\"],\"dimensions\":[1],\"domain\":\"RBDmodel/L2-L3 FE readings/L2-L3 FE Simscape\",\"lineColor\":\"#fe330a\",\"port\":1,\"sid\":[\"\"],\"signalID\":1888,\"signalName\":\"L2-L3 FE Simscape Rotation\"},\"type\":\"RecordBlkView.Signal\",\"uuid\":\"74e04804-8fe0-4986-8570-2130713f6701\"},{\"content\":{\"blockPath\":[\"RBDmodel/L2-L3 FE readings/L2-L3 FE Simscape\"],\"dimensions\":[1],\"domain\":\"RBDmodel/L2-L3 FE readings/L2-L3 FE Simscape\",\"lineColor\":\"#22b573\",\"port\":2,\"sid\":[\"\"],\"signalID\":1892,\"signalName\":\"L2-L3 FE Simscape Moment\"},\"type\":\"RecordBlkView.Signal\",\"uuid\":\"afa977c3-f7f3-4479-b4e8-b42df805f44b\"}]},\"type\":\"RecordBlkView.InputSignals\",\"uuid\":\"d0d120ea-f189-4cd8-a4da-cbfdd5b90160\"}],\"packageUris\":[\"http://schema.mathworks.com/mf0/streamout_blocks/R2020a\"],\"version\":\"1.0\"}"  VisualizationBindings="{\"xyplotplugin\":{\"info\":[{\"series\":[],\"subplotID\":1}]}}"  CompatibilityTag=XY
  wires:
  L2-L3 FE Simscape Rotation/1 -> L2-L3 FE Simscape/1, L2-L3 FE Rotation/1
  L2-L3 FE Simscape Moment/1 -> L2-L3 FE Simscape/2, L2-L3 FE Moment/1

== system RBDmodel_unprotected/L2-L3 LB readings ==
  L2-L3 LB Simscape Rotation : Inport
  L2-L3 LB Simscape Moment : Inport  Port=2
  L2-L3 LB Moment : Scope
  L2-L3 LB Rotation : Scope
  L2-L3 LB Simscape : Record  FileSettingsInternal="{\"entries\":[{\"content\":{\"excelSettings\":{\"content\":{},\"type\":\"Streamout.ExcelSettings\"}},\"type\":\"Streamout.FileSettingStorage\",\"uuid\":\"878bef31-d79f-4083-a205-bcf592f6bcb0\"}],\"packageUris\":[\"http://schema.mathworks.com/mf0/streamout_blocks/R2020a\"],\"version\":\"1.0\"}"  Layout=[1 1]  SignalsInternal="{\"entries\":[{\"content\":{\"signals\":[{\"content\":{\"blockPath\":[\"RBDmodel/L2-L3 LB readings/L2-L3 LB Simscape\"],\"dimensions\":[1],\"domain\":\"RBDmodel/L2-L3 LB readings/L2-L3 LB Simscape\",\"lineColor\":\"#0072bd\",\"port\":1,\"sid\":[\"\"],\"signalID\":1896,\"signalName\":\"L2-L3 LB Simscape Rotation\"},\"type\":\"RecordBlkView.Signal\",\"uuid\":\"b30462aa-01a8-4be7-8ad7-812217bf6dfe\"},{\"content\":{\"blockPath\":[\"RBDmodel/L2-L3 LB readings/L2-L3 LB Simscape\"],\"dimensions\":[1],\"domain\":\"RBDmodel/L2-L3 LB readings/L2-L3 LB Simscape\",\"lineColor\":\"#d95319\",\"port\":2,\"sid\":[\"\"],\"signalID\":1900,\"signalName\":\"L2-L3 LB Simscape Moment\"},\"type\":\"RecordBlkView.Signal\",\"uuid\":\"9166c31e-8a27-4614-bed1-8ee03d89d5cf\"}]},\"type\":\"RecordBlkView.InputSignals\",\"uuid\":\"78127789-2375-492c-b5a9-32fb6a6e66a6\"}],\"packageUris\":[\"http://schema.mathworks.com/mf0/streamout_blocks/R2020a\"],\"version\":\"1.0\"}"  VisualizationBindings="{\"xyplotplugin\":{\"info\":[{\"series\":[],\"subplotID\":1}]}}"  CompatibilityTag=XY
  wires:
  L2-L3 LB Simscape Rotation/1 -> L2-L3 LB Simscape/1, L2-L3 LB Rotation/1
  L2-L3 LB Simscape Moment/1 -> L2-L3 LB Simscape/2, L2-L3 LB Moment/1

== system RBDmodel_unprotected/L3-L4 AR readings ==
  L3-L4 AR Simscape Rotation : Inport
  L3-L4 AR Simscape Moment : Inport  Port=2
  L3-L4 AR Moment : Scope
  L3-L4 AR Rotation : Scope
  L3-L4 AR Simscape : Record  FileSettingsInternal="{\"entries\":[{\"content\":{\"excelSettings\":{\"content\":{},\"type\":\"Streamout.ExcelSettings\"}},\"type\":\"Streamout.FileSettingStorage\",\"uuid\":\"ed70d5eb-48f6-433c-a28d-6e368c0f1543\"}],\"packageUris\":[\"http://schema.mathworks.com/mf0/streamout_blocks/R2020a\"],\"version\":\"1.0\"}"  Layout=[1 1]  SignalsInternal="{\"entries\":[{\"content\":{\"signals\":[{\"content\":{\"blockPath\":[\"RBDmodel/L3-L4 AR readings/L3-L4 AR Simscape\"],\"dimensions\":[1],\"domain\":\"RBDmodel/L3-L4 AR readings/L3-L4 AR Simscape\",\"lineColor\":\"#edb120\",\"port\":1,\"sid\":[\"\"],\"signalID\":1904,\"signalName\":\"L3-L4 AR Simscape Rotation\"},\"type\":\"RecordBlkView.Signal\",\"uuid\":\"2e09b9e4-f336-4963-89c3-e1dc9a948c10\"},{\"content\":{\"blockPath\":[\"RBDmodel/L3-L4 AR readings/L3-L4 AR Simscape\"],\"dimensions\":[1],\"domain\":\"RBDmodel/L3-L4 AR readings/L3-L4 AR Simscape\",\"lineColor\":\"#7e2f8e\",\"port\":2,\"sid\":[\"\"],\"signalID\":1908,\"signalName\":\"L3-L4 AR Simscape Moment\"},\"type\":\"RecordBlkView.Signal\",\"uuid\":\"3f04ecc8-97e1-45fd-8bde-07a328216503\"}]},\"type\":\"RecordBlkView.InputSignals\",\"uuid\":\"85a4f14a-2379-4227-9d25-fba8887534b6\"}],\"packageUris\":[\"http://schema.mathworks.com/mf0/streamout_blocks/R2020a\"],\"version\":\"1.0\"}"  VisualizationBindings="{\"xyplotplugin\":{\"info\":[{\"series\":[],\"subplotID\":1}]}}"  CompatibilityTag=XY
  wires:
  L3-L4 AR Simscape Rotation/1 -> L3-L4 AR Simscape/1, L3-L4 AR Rotation/1
  L3-L4 AR Simscape Moment/1 -> L3-L4 AR Simscape/2, L3-L4 AR Moment/1

== system RBDmodel_unprotected/L3-L4 FE readings ==
  L3-L4 FE Simscape Rotation : Inport
  L3-L4 FE Simscape Moment : Inport  Port=2
  L3-L4 FE Moment : Scope
  L3-L4 FE Rotation : Scope
  L3-L4 FE Simscape : Record  FileSettingsInternal="{\"entries\":[{\"content\":{\"excelSettings\":{\"content\":{},\"type\":\"Streamout.ExcelSettings\"}},\"type\":\"Streamout.FileSettingStorage\",\"uuid\":\"1aee1af9-8fc8-4730-a4e0-7af1bcb30507\"}],\"packageUris\":[\"http://schema.mathworks.com/mf0/streamout_blocks/R2020a\"],\"version\":\"1.0\"}"  Layout=[1 1]  SignalsInternal="{\"entries\":[{\"content\":{\"signals\":[{\"content\":{\"blockPath\":[\"RBDmodel/L3-L4 FE readings/L3-L4 FE Simscape\"],\"dimensions\":[1],\"domain\":\"RBDmodel/L3-L4 FE readings/L3-L4 FE Simscape\",\"lineColor\":\"#77ac30\",\"port\":1,\"sid\":[\"\"],\"signalID\":1912,\"signalName\":\"L3-L4 FE Simscape Rotation\"},\"type\":\"RecordBlkView.Signal\",\"uuid\":\"1bd73186-cb2d-40ad-b4cf-d15f31148705\"},{\"content\":{\"blockPath\":[\"RBDmodel/L3-L4 FE readings/L3-L4 FE Simscape\"],\"dimensions\":[1],\"domain\":\"RBDmodel/L3-L4 FE readings/L3-L4 FE Simscape\",\"lineColor\":\"#4dbeee\",\"port\":2,\"sid\":[\"\"],\"signalID\":1916,\"signalName\":\"L3-L4 FE Simscape Moment\"},\"type\":\"RecordBlkView.Signal\",\"uuid\":\"26886949-396b-49a8-a57a-d4002349d880\"}]},\"type\":\"RecordBlkView.InputSignals\",\"uuid\":\"9a9d9143-ab15-4628-ad81-34444a67b9a3\"}],\"packageUris\":[\"http://schema.mathworks.com/mf0/streamout_blocks/R2020a\"],\"version\":\"1.0\"}"  VisualizationBindings="{\"xyplotplugin\":{\"info\":[{\"series\":[],\"subplotID\":1}]}}"  CompatibilityTag=XY
  wires:
  L3-L4 FE Simscape Rotation/1 -> L3-L4 FE Simscape/1, L3-L4 FE Rotation/1
  L3-L4 FE Simscape Moment/1 -> L3-L4 FE Simscape/2, L3-L4 FE Moment/1

== system RBDmodel_unprotected/L3-L4 LB readings ==
  L3-L4 LB Simscape Rotation : Inport
  L3-L4 LB Simscape Moment : Inport  Port=2
  L3-L4 LB Moment : Scope
  L3-L4 LB Rotation : Scope
  L3-L4 LB Simscape : Record  FileSettingsInternal="{\"entries\":[{\"content\":{\"excelSettings\":{\"content\":{},\"type\":\"Streamout.ExcelSettings\"}},\"type\":\"Streamout.FileSettingStorage\",\"uuid\":\"0635f9a3-32cd-448c-ad9c-6f4c32d19c01\"}],\"packageUris\":[\"http://schema.mathworks.com/mf0/streamout_blocks/R2020a\"],\"version\":\"1.0\"}"  Layout=[1 1]  SignalsInternal="{\"entries\":[{\"content\":{\"signals\":[{\"content\":{\"blockPath\":[\"RBDmodel/L3-L4 LB readings/L3-L4 LB Simscape\"],\"dimensions\":[1],\"domain\":\"RBDmodel/L3-L4 LB readings/L3-L4 LB Simscape\",\"lineColor\":\"#a2142f\",\"port\":1,\"sid\":[\"\"],\"signalID\":1920,\"signalName\":\"L3-L4 LB Simscape Rotation\"},\"type\":\"RecordBlkView.Signal\",\"uuid\":\"c40a0175-9443-44c2-b36e-22a631689830\"},{\"content\":{\"blockPath\":[\"RBDmodel/L3-L4 LB readings/L3-L4 LB Simscape\"],\"dimensions\":[1],\"domain\":\"RBDmodel/L3-L4 LB readings/L3-L4 LB Simscape\",\"lineColor\":\"#139fff\",\"port\":2,\"sid\":[\"\"],\"signalID\":1924,\"signalName\":\"L3-L4 LB Simscape Moment\"},\"type\":\"RecordBlkView.Signal\",\"uuid\":\"c8b7a6d4-b260-4e69-bd6e-bf9f5c2c32d8\"}]},\"type\":\"RecordBlkView.InputSignals\",\"uuid\":\"633aeb3b-d9d2-49fd-9549-3c06cd711e5b\"}],\"packageUris\":[\"http://schema.mathworks.com/mf0/streamout_blocks/R2020a\"],\"version\":\"1.0\"}"  VisualizationBindings="{\"xyplotplugin\":{\"info\":[{\"series\":[],\"subplotID\":1}]}}"  CompatibilityTag=XY
  wires:
  L3-L4 LB Simscape Rotation/1 -> L3-L4 LB Simscape/1, L3-L4 LB Rotation/1
  L3-L4 LB Simscape Moment/1 -> L3-L4 LB Simscape/2, L3-L4 LB Moment/1

== system RBDmodel_unprotected/L4-L5 AR readings ==
  L4-L5 AR Simscape Rotation : Inport
  L4-L5 AR Simscape Moment : Inport  Port=2
  L4-L5 AR Moment : Scope
  L4-L5 AR Rotation : Scope
  L4-L5 AR Simscape : Record  FileSettingsInternal="{\"entries\":[{\"content\":{\"excelSettings\":{\"content\":{},\"type\":\"Streamout.ExcelSettings\"}},\"type\":\"Streamout.FileSettingStorage\",\"uuid\":\"f3f48697-9fec-488e-8242-af8fd6f53404\"}],\"packageUris\":[\"http://schema.mathworks.com/mf0/streamout_blocks/R2020a\"],\"version\":\"1.0\"}"  Layout=[1 1]  SignalsInternal="{\"entries\":[{\"content\":{\"signals\":[{\"content\":{\"blockPath\":[\"RBDmodel/L4-L5 AR readings/L4-L5 AR Simscape\"],\"dimensions\":[1],\"domain\":\"RBDmodel/L4-L5 AR readings/L4-L5 AR Simscape\",\"lineColor\":\"#ff6929\",\"port\":1,\"sid\":[\"\"],\"signalID\":1928,\"signalName\":\"L4-L5 AR Simscape Rotation\"},\"type\":\"RecordBlkView.Signal\",\"uuid\":\"0350062c-a4d9-41c6-8ca7-2a3caaa77f36\"},{\"content\":{\"blockPath\":[\"RBDmodel/L4-L5 AR readings/L4-L5 AR Simscape\"],\"dimensions\":[1],\"domain\":\"RBDmodel/L4-L5 AR readings/L4-L5 AR Simscape\",\"lineColor\":\"#b746ff\",\"port\":2,\"sid\":[\"\"],\"signalID\":1932,\"signalName\":\"L4-L5 AR Simscape Moment\"},\"type\":\"RecordBlkView.Signal\",\"uuid\":\"46071015-32b0-42cf-83ac-dafe7b09c9cb\"}]},\"type\":\"RecordBlkView.InputSignals\",\"uuid\":\"fd7b49f8-5f70-4eef-b375-f5e6bfb5c7dd\"}],\"packageUris\":[\"http://schema.mathworks.com/mf0/streamout_blocks/R2020a\"],\"version\":\"1.0\"}"  VisualizationBindings="{\"xyplotplugin\":{\"info\":[{\"series\":[],\"subplotID\":1}]}}"  CompatibilityTag=XY
  wires:
  L4-L5 AR Simscape Moment/1 -> L4-L5 AR Simscape/2, L4-L5 AR Moment/1
  L4-L5 AR Simscape Rotation/1 -> L4-L5 AR Simscape/1, L4-L5 AR Rotation/1

== system RBDmodel_unprotected/L4-L5 FE readings ==
  L4-L5 FE Simscape Rotation : Inport
  L4-L5 FE Simscape Moment : Inport  Port=2
  L4-L5 FE Moment : Scope
  L4-L5 FE Rotation : Scope
  L4-L5 FE Simscape : Record  FileSettingsInternal="{\"entries\":[{\"content\":{\"excelSettings\":{\"content\":{},\"type\":\"Streamout.ExcelSettings\"}},\"type\":\"Streamout.FileSettingStorage\",\"uuid\":\"e890ad54-8517-454b-a26e-30f954ae6c08\"}],\"packageUris\":[\"http://schema.mathworks.com/mf0/streamout_blocks/R2020a\"],\"version\":\"1.0\"}"  Layout=[1 1]  SignalsInternal="{\"entries\":[{\"content\":{\"signals\":[{\"content\":{\"blockPath\":[\"RBDmodel/L4-L5 FE readings/L4-L5 FE Simscape\"],\"dimensions\":[1],\"domain\":\"RBDmodel/L4-L5 FE readings/L4-L5 FE Simscape\",\"lineColor\":\"#64d413\",\"port\":1,\"sid\":[\"\"],\"signalID\":1936,\"signalName\":\"L4-L5 FE Simscape Rotation\"},\"type\":\"RecordBlkView.Signal\",\"uuid\":\"0bb19487-c07b-40cb-bef9-7f984b0ccd07\"},{\"content\":{\"blockPath\":[\"RBDmodel/L4-L5 FE readings/L4-L5 FE Simscape\"],\"dimensions\":[1],\"domain\":\"RBDmodel/L4-L5 FE readings/L4-L5 FE Simscape\",\"lineColor\":\"#ff13a6\",\"port\":2,\"sid\":[\"\"],\"signalID\":1940,\"signalName\":\"L4-L5 FE Simscape Moment\"},\"type\":\"RecordBlkView.Signal\",\"uuid\":\"5f778a4c-23ce-4734-9441-2f8b8778c402\"}]},\"type\":\"RecordBlkView.InputSignals\",\"uuid\":\"c9c84afd-6e6d-4d5e-8181-f3e7990edce0\"}],\"packageUris\":[\"http://schema.mathworks.com/mf0/streamout_blocks/R2020a\"],\"version\":\"1.0\"}"  VisualizationBindings="{\"xyplotplugin\":{\"info\":[{\"series\":[],\"subplotID\":1}]}}"  CompatibilityTag=XY
  wires:
  L4-L5 FE Simscape Rotation/1 -> L4-L5 FE Simscape/1, L4-L5 FE Rotation/1
  L4-L5 FE Simscape Moment/1 -> L4-L5 FE Simscape/2, L4-L5 FE Moment/1

== system RBDmodel_unprotected/L4-L5 LB readings ==
  L4-L5 LB Simscape Rotation : Inport
  L4-L5 LB Simscape Moment : Inport  Port=2
  L4-L5 LB Moment : Scope
  L4-L5 LB Rotation : Scope
  L4-L5 LB Simscape : Record  FileSettingsInternal="{\"entries\":[{\"content\":{\"excelSettings\":{\"content\":{},\"type\":\"Streamout.ExcelSettings\"}},\"type\":\"Streamout.FileSettingStorage\",\"uuid\":\"7ca7c28a-7266-4226-beab-37365eead35d\"}],\"packageUris\":[\"http://schema.mathworks.com/mf0/streamout_blocks/R2020a\"],\"version\":\"1.0\"}"  Layout=[1 1]  SignalsInternal="{\"entries\":[{\"content\":{\"signals\":[{\"content\":{\"blockPath\":[\"RBDmodel/L4-L5 LB readings/L4-L5 LB Simscape\"],\"dimensions\":[1],\"domain\":\"RBDmodel/L4-L5 LB readings/L4-L5 LB Simscape\",\"lineColor\":\"#fe330a\",\"port\":1,\"sid\":[\"\"],\"signalID\":1944,\"signalName\":\"L4-L5 LB Simscape Rotation\"},\"type\":\"RecordBlkView.Signal\",\"uuid\":\"dbfb82ae-8e44-4961-aa1a-c4b4275756eb\"},{\"content\":{\"blockPath\":[\"RBDmodel/L4-L5 LB readings/L4-L5 LB Simscape\"],\"dimensions\":[1],\"domain\":\"RBDmodel/L4-L5 LB readings/L4-L5 LB Simscape\",\"lineColor\":\"#22b573\",\"port\":2,\"sid\":[\"\"],\"signalID\":1948,\"signalName\":\"L4-L5 LB Simscape Moment\"},\"type\":\"RecordBlkView.Signal\",\"uuid\":\"4ba4bcdd-f88c-4ee8-946a-951db70efdad\"}]},\"type\":\"RecordBlkView.InputSignals\",\"uuid\":\"a679c17f-a3cd-419e-9af5-5763557a9d40\"}],\"packageUris\":[\"http://schema.mathworks.com/mf0/streamout_blocks/R2020a\"],\"version\":\"1.0\"}"  VisualizationBindings="{\"xyplotplugin\":{\"info\":[{\"series\":[],\"subplotID\":1}]}}"  CompatibilityTag=XY
  wires:
  L4-L5 LB Simscape Moment/1 -> L4-L5 LB Simscape/2, L4-L5 LB Moment/1
  L4-L5 LB Simscape Rotation/1 -> L4-L5 LB Simscape/1, L4-L5 LB Rotation/1

== system RBDmodel_unprotected/L5-S1 AR readings ==
  L5-S1 AR Simscape Rotation : Inport
  L5-S1 AR Simscape Moment : Inport  Port=2
  L5-S1 AR Moment : Scope
  L5-S1 AR Rotation : Scope
  L5-S1 AR Simscape : Record  FileSettingsInternal="{\"entries\":[{\"content\":{\"excelSettings\":{\"content\":{},\"type\":\"Streamout.ExcelSettings\"}},\"type\":\"Streamout.FileSettingStorage\",\"uuid\":\"27abd9e2-1d5b-4eb3-b760-2ba53000626f\"}],\"packageUris\":[\"http://schema.mathworks.com/mf0/streamout_blocks/R2020a\"],\"version\":\"1.0\"}"  Layout=[1 1]  SignalsInternal="{\"entries\":[{\"content\":{\"signals\":[{\"content\":{\"blockPath\":[\"RBDmodel/L5-S1 AR readings/L5-S1 AR Simscape\"],\"dimensions\":[1],\"domain\":\"RBDmodel/L5-S1 AR readings/L5-S1 AR Simscape\",\"lineColor\":\"#0072bd\",\"port\":1,\"sid\":[\"\"],\"signalID\":1952,\"signalName\":\"L5-S1 AR Simscape Rotation\"},\"type\":\"RecordBlkView.Signal\",\"uuid\":\"b7da56bc-79ab-4a5c-8813-8a68960312d4\"},{\"content\":{\"blockPath\":[\"RBDmodel/L5-S1 AR readings/L5-S1 AR Simscape\"],\"dimensions\":[1],\"domain\":\"RBDmodel/L5-S1 AR readings/L5-S1 AR Simscape\",\"lineColor\":\"#d95319\",\"port\":2,\"sid\":[\"\"],\"signalID\":1956,\"signalName\":\"L5-S1 AR Simscape Moment\"},\"type\":\"RecordBlkView.Signal\",\"uuid\":\"92ce0386-1be2-4a43-8e23-40db634d2efc\"}]},\"type\":\"RecordBlkView.InputSignals\",\"uuid\":\"d489a2cb-afb8-41d4-af53-4721548de882\"}],\"packageUris\":[\"http://schema.mathworks.com/mf0/streamout_blocks/R2020a\"],\"version\":\"1.0\"}"  VisualizationBindings="{\"xyplotplugin\":{\"info\":[{\"series\":[],\"subplotID\":1}]}}"  CompatibilityTag=XY
  wires:
  L5-S1 AR Simscape Rotation/1 -> L5-S1 AR Simscape/1, L5-S1 AR Rotation/1
  L5-S1 AR Simscape Moment/1 -> L5-S1 AR Simscape/2, L5-S1 AR Moment/1

== system RBDmodel_unprotected/L5-S1 FE readings ==
  L5-S1 FE Simscape Rotation : Inport
  L5-S1 FE Simscape Moment : Inport  Port=2
  L5-S1 FE M-R : Record  FileSettingsInternal="{\"entries\":[{\"content\":{\"excelSettings\":{\"content\":{},\"type\":\"Streamout.ExcelSettings\"}},\"type\":\"Streamout.FileSettingStorage\",\"uuid\":\"e01f2ac1-1811-44c6-a984-bb03a8f3b2a8\"}],\"packageUris\":[\"http://schema.mathworks.com/mf0/streamout_blocks/R2020a\"],\"version\":\"1.0\"}"  Layout=[1 1]  SignalsInternal="{\"entries\":[{\"content\":{\"signals\":[{\"content\":{\"blockPath\":[\"RBDmodel/L5-S1 FE readings/L5-S1 FE M-R\"],\"dimensions\":[1],\"domain\":\"RBDmodel/L5-S1 FE readings/L5-S1 FE M-R\",\"lineColor\":\"#edb120\",\"port\":1,\"sid\":[\"\"],\"signalID\":1960,\"signalName\":\"L5-S1 FE Simscape Rotation\"},\"type\":\"RecordBlkView.Signal\",\"uuid\":\"e51a3b7e-f8bc-4b83-9b0b-735875f99908\"},{\"content\":{\"blockPath\":[\"RBDmodel/L5-S1 FE readings/L5-S1 FE M-R\"],\"dimensions\":[1],\"domain\":\"RBDmodel/L5-S1 FE readings/L5-S1 FE M-R\",\"lineColor\":\"#7e2f8e\",\"port\":2,\"sid\":[\"\"],\"signalID\":1964,\"signalName\":\"L5-S1 FE Simscape Moment\"},\"type\":\"RecordBlkView.Signal\",\"uuid\":\"4c8f9aee-fd2c-486d-b444-e72e110198a2\"}]},\"type\":\"RecordBlkView.InputSignals\",\"uuid\":\"6d7d3d56-862b-4958-8df6-064b03a20ebb\"}],\"packageUris\":[\"http://schema.mathworks.com/mf0/streamout_blocks/R2020a\"],\"version\":\"1.0\"}"  VisualizationBindings="{\"xyplotplugin\":{\"info\":[{\"series\":[],\"subplotID\":1}]}}"  CompatibilityTag=XY
  L5-S1 FE Moment : Scope
  L5-S1 FE Rot : Scope
  wires:
  L5-S1 FE Simscape Rotation/1 -> L5-S1 FE M-R/1, L5-S1 FE Rot/1
  L5-S1 FE Simscape Moment/1 -> L5-S1 FE M-R/2, L5-S1 FE Moment/1

== system RBDmodel_unprotected/L5-S1 LB readings ==
  L5-S1 LB Simscape Rotation : Inport
  L5-S1 LB Simscape Moment : Inport  Port=2
  L5-S1 LB Moment : Scope
  L5-S1 LB Rotation : Scope
  L5-S1 LB Simscape : Record  FileSettingsInternal="{\"entries\":[{\"content\":{\"excelSettings\":{\"content\":{},\"type\":\"Streamout.ExcelSettings\"}},\"type\":\"Streamout.FileSettingStorage\",\"uuid\":\"f04f4f76-9a90-4b9c-a34a-ac02ee8fff49\"}],\"packageUris\":[\"http://schema.mathworks.com/mf0/streamout_blocks/R2020a\"],\"version\":\"1.0\"}"  Layout=[1 1]  SignalsInternal="{\"entries\":[{\"content\":{\"signals\":[{\"content\":{\"blockPath\":[\"RBDmodel/L5-S1 LB readings/L5-S1 LB Simscape\"],\"dimensions\":[1],\"domain\":\"RBDmodel/L5-S1 LB readings/L5-S1 LB Simscape\",\"lineColor\":\"#77ac30\",\"port\":1,\"sid\":[\"\"],\"signalID\":1968,\"signalName\":\"L5-S1 LB Simscape Rotation\"},\"type\":\"RecordBlkView.Signal\",\"uuid\":\"dfd019cb-2756-4367-8e0e-193d048e5e50\"},{\"content\":{\"blockPath\":[\"RBDmodel/L5-S1 LB readings/L5-S1 LB Simscape\"],\"dimensions\":[1],\"domain\":\"RBDmodel/L5-S1 LB readings/L5-S1 LB Simscape\",\"lineColor\":\"#4dbeee\",\"port\":2,\"sid\":[\"\"],\"signalID\":1972,\"signalName\":\"L5-S1 LB Simscape Moment\"},\"type\":\"RecordBlkView.Signal\",\"uuid\":\"7a169e80-2d94-4c37-a72a-8f2aed7f5543\"}]},\"type\":\"RecordBlkView.InputSignals\",\"uuid\":\"6aecad3e-f9c0-458d-9151-f882adfede50\"}],\"packageUris\":[\"http://schema.mathworks.com/mf0/streamout_blocks/R2020a\"],\"version\":\"1.0\"}"  VisualizationBindings="{\"xyplotplugin\":{\"info\":[{\"series\":[],\"subplotID\":1}]}}"  CompatibilityTag=XY
  wires:
  L5-S1 LB Simscape Moment/1 -> L5-S1 LB Simscape/2, L5-S1 LB Moment/1
  L5-S1 LB Simscape Rotation/1 -> L5-S1 LB Simscape/1, L5-S1 LB Rotation/1

== system RBDmodel_unprotected/Left ITL Readings ==
  In1 : Inport
  In2 : Inport  Port=2
  In3 : Inport  Port=3
  In4 : Inport  Port=4
  In5 : Inport  Port=5
  Left L1-L2 ITL force : Scope
  Left L2-L3 ITL force : Scope
  Left L4-L5 ITL force : Scope
  Left L5-S1 ITL force : Scope
  Let L3-L4 ITL force : Scope
  wires:
  In4/1 -> Left L4-L5 ITL force/1
  In1/1 -> Left L1-L2 ITL force/1
  In5/1 -> Let L3-L4 ITL force/1
  In3/1 -> Left L5-S1 ITL force/1
  In2/1 -> Left L2-L3 ITL force/1

== system RBDmodel_unprotected/Muscle force inputs ==
  Area in mm^2 : Constant  Value=26819
  Constant : Constant  Value=100000
  Display : Display
  Divide : Product  Inputs=**/
  IAP in Pascals : Constant  Value=IAP_Pa
  Left Abdominal Muscle Force : Constant  Value=-Left_RA
  Left Back Muscle Force : Constant  Value=-Left_MF
  Left Transverse1 Muscle Force : Constant  Value=-Left_IO
  Left Transverse2 Muscle Force : Constant  Value=-Left_EO
  Right Abdominal Muscle Force : Constant  Value=-Right_RA
  Right Back Muscle Force : Constant  Value=-Right_MF
  Right Transverse1 Muscle Force : Constant  Value=-Right_IO
  Right Transverse2 Muscle Force : Constant  Value=-Right_EO
  Scope{1..8} (8 alike) : Scope
  Sum of Square of Forces : MATLAB Function  TreatAsAtomicUnit=on
  Right RA : Outport
  Left RA : Outport  Port=2
  Right MF : Outport  Port=3
  Left MF : Outport  Port=4
  Right IO : Outport  Port=5
  Right EO : Outport  Port=6
  Left IO : Outport  Port=7
  Left EO : Outport  Port=8
  wires:
  Left Transverse2 Muscle Force/1 -> Left EO/1, Scope8/1, Sum of Square of Forces/8(F8)  "LeftTransverse2MuscleForce"
  Left Abdominal Muscle Force/1 -> Left RA/1, Scope2/1, Sum of Square of Forces/2(F2)  "LeftAbdominalMuscleForce"
  Sum of Square of Forces/1(SumofSquareofForces) -> Display/1  "SumofSquareofForces"
  Area in mm^2/1 -> Divide/2
  Left Back Muscle Force/1 -> Sum of Square of Forces/4(F4), Left MF/1, Scope4/1  "LeftBackMuscleForce"
  Divide/1 -> Sum of Square of Forces/9(IAP)
  Left Transverse1 Muscle Force/1 -> Left IO/1, Scope7/1, Sum of Square of Forces/6(F6)  "LeftTransverse1MuscleForce"
  Right Abdominal Muscle Force/1 -> Right RA/1, Scope1/1, Sum of Square of Forces/1(F1)  "RightAbdominalMuscleForce"
  Right Back Muscle Force/1 -> Right MF/1, Scope3/1, Sum of Square of Forces/3(F3)  "RightBackMuscleForce"
  Right Transverse2 Muscle Force/1 -> Right EO/1, Scope6/1, Sum of Square of Forces/5(F5)  "RightTransverse2MuscleForce"
  Right Transverse1 Muscle Force/1 -> Right IO/1, Scope5/1, Sum of Square of Forces/7(F7)  "RightTransverse1MuscleForce"
  IAP in Pascals/1 -> Divide/1
  Constant/1 -> Divide/3

== system RBDmodel_unprotected/Plumbline readings ==
  x : Inport
  y : Inport  Port=2
  z : Inport  Port=3
  Check X Bounds : checkpacklib/Check Custom Bounds  InstantiateOnLoad=on  enabled=off  stopWhenAssertionFail=off  export=off  ViewDlgPos=[983.4 172.2 510.4 379.2]  OpenViewOnLoad=off  LaunchViewOnOpen=off  TimeUnits=seconds  EnableUpperBound=on  UpperBoundTimes=[0 3]  UpperBoundAmplitudes=[2 2];  EnableLowerBound=on  LowerBoundTimes=[0 3]  LowerBoundAmplitudes=[-2 -2]
      settings: LibrarySourceBlock=sdolib/Signal Constraints/Check Custom Bounds
  Check Y Bounds : checkpacklib/Check Custom Bounds  InstantiateOnLoad=on  enabled=off  stopWhenAssertionFail=off  export=off  ViewDlgPos=[509 222 510 390]  OpenViewOnLoad=off  LaunchViewOnOpen=off  TimeUnits=seconds  EnableUpperBound=on  UpperBoundTimes=[0 3]  UpperBoundAmplitudes=[2 2];  EnableLowerBound=on  LowerBoundTimes=[0 3]  LowerBoundAmplitudes=[-2 -2]
      settings: LibrarySourceBlock=sdolib/Signal Constraints/Check Custom Bounds
  Plumbline X distance (cm) : Display
  Plumbline Y distance (cm) : Display
  Plumbline Z distance (cm) : Display
  T1 plumbline coordinates : Scope  NumInputPorts=3
  wires:
  x/1 -> Plumbline X distance (cm)/1, Check X Bounds/1, T1 plumbline coordinates/1
  z/1 -> Plumbline Z distance (cm)/1, T1 plumbline coordinates/3
  y/1 -> Plumbline Y distance (cm)/1, Check Y Bounds/1, T1 plumbline coordinates/2
